simulink model "ASK_nc"  (R2020a)
settings: Solver=VariableStepDiscrete  StartTime=0.0  StopTime=tsim  RelTol=1e-3
values from neighbouring files (symbols this model uses):
  Ac = 1    [init_vars.m]
  B = rb    (= 1000)    [init_vars.m]
  fc = 10e3    (= 10000)    [init_vars.m]
  fs = spb * rb    (= 100000)    [init_vars.m]
  lim = 0.5/2    (= 0.25)    [parte3ASK.m]    (also in parte3BPSK.m = 0; parte4.m)
  rb = 1e3    (= 1000)    [init_vars.m]
  rng_seed = 5    [init_vars.m]
  spb = 100    [init_vars.m]
undefined symbols (not defined in the file or in its folder): fdesignblkfcn, gcbh
libraries: dspswit3 x2, commrandsrc3 x1, commchan3 x1, dspsigops x1, dspfdesign x1
settings Model: Creator=pedro  LastModifiedBy=pedro

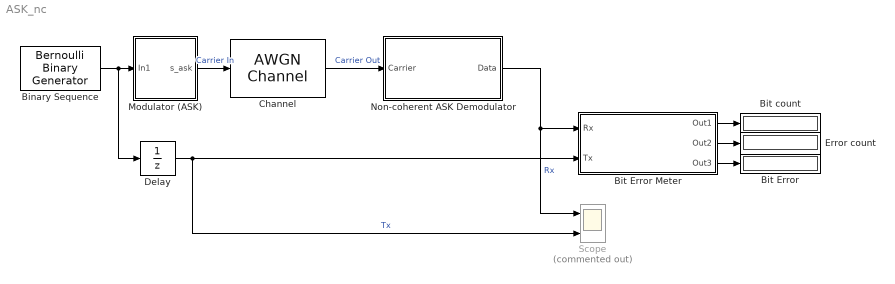
== system ASK_nc ==
  Binary Sequence : commrandsrc3/Bernoulli Binary Generator  ProbabilityOfZero=0.5  SeedSource=Parameter  Seed=rng_seed  SampleTime=1/rb  SamplesPerFrame=1  OutputDataType=double  SimulateUsing=Interpreted execution
  Bit Error : Display
  Bit Error Meter : Subsystem
  Bit count : Display
  Channel : commchan3/AWGN Channel  InputProcessing=Columns as channels (frame based)  seed=rng_seed  noiseMode=Variance from mask  EbNodB=10  EsNodB=10  SNRdB=10  bitsPerSym=1  Ps=1  Tsym=1  variance=sigmaquadrado
  Delay : UnitDelay  SampleTime=1/rb  HasFrameUpgradeWarning=on
  Error count : Display
  Modulator (ASK) : Subsystem
  Non-coherent ASK Demodulator : Subsystem
  Scope : Scope  Commented=on  NumInputPorts=2
  wires:
  Bit Error Meter/1(Out1) -> Bit count/1
  Bit Error Meter/2(Out2) -> Error count/1
  Delay/1 -> Scope/2, Bit Error Meter/2(Tx)  "Tx"
  Binary Sequence/1 -> Delay/1, Modulator (ASK)/1(In1)
  Bit Error Meter/3(Out3) -> Bit Error/1
  Modulator (ASK)/1(s_ask) -> Channel/1  "Carrier In"
  Channel/1 -> Non-coherent ASK Demodulator/1(Carrier)  "Carrier Out"
  Non-coherent ASK Demodulator/1(Data) -> Bit Error Meter/1(Rx), Scope/1  "Rx"

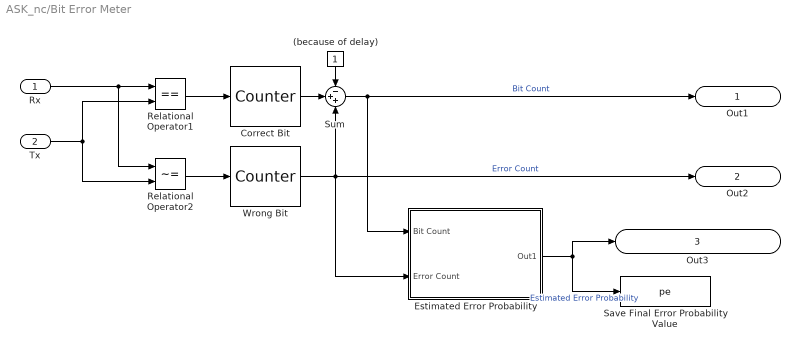
== system ASK_nc/Bit Error Meter ==
  Rx : Inport
  Tx : Inport  Port=2
  (because of delay) : Constant
  Correct Bit : dspswit3/Counter  Direction=Up  CountEvent=Non-zero sample  CounterSize=32 bits  MaxCount=255  InitialCount=0  Output=Count  HitValue=32  ResetInput=off  SamplesPerFrame=1  Ts=1  CntDtype=uint32  HitDtype=Logical
  Estimated Error Probability : Subsystem
  Relational Operator1 : RelationalOperator  Operator===  OutDataTypeStr=boolean  RndMeth=Simplest
  Relational Operator2 : RelationalOperator  Operator=~=  OutDataTypeStr=boolean  RndMeth=Simplest
  Save Final Error Probability Value : ToWorkspace  VariableName=pe  SampleTime=-1
      settings: MaxDataPoints=1
  Sum : Sum  Inputs=-++
  Wrong Bit : dspswit3/Counter  Direction=Up  CountEvent=Non-zero sample  CounterSize=32 bits  MaxCount=255  InitialCount=0  Output=Count  HitValue=32  ResetInput=off  SamplesPerFrame=1  Ts=1  CntDtype=uint32  HitDtype=Logical
  Out1 : Outport
  Out2 : Outport  Port=2
  Out3 : Outport  Port=3
  wires:
  Relational Operator1/1 -> Correct Bit/1
  Correct Bit/1 -> Sum/2
  Rx/1 -> Relational Operator2/1, Relational Operator1/1
  Relational Operator2/1 -> Wrong Bit/1
  Sum/1 -> Estimated Error Probability/1(Bit Count), Out1/1  "Bit Count"
  Tx/1 -> Relational Operator2/2, Relational Operator1/2
  Wrong Bit/1 -> Estimated Error Probability/2(Error Count), Sum/3, Out2/1  "Error Count"
  (because of delay)/1 -> Sum/1
  Estimated Error Probability/1(Out1) -> Save Final Error Probability Value/1, Out3/1  "Estimated Error Probability"

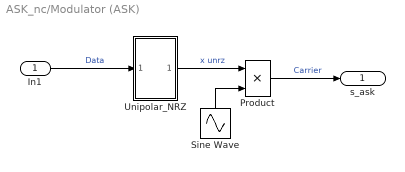
== system ASK_nc/Modulator (ASK) ==
  In1 : Inport
  Product : Product
  Sine Wave : Sin  Amplitude=Ac  Frequency=2*pi*fc  SampleTime=1/fs
  Unipolar_NRZ : Subsystem  mask(unipolar_nrz){Rb=rb, Spb=spb}
      mask prompts: Rb "Binary Data Rate"; Spb "Samples per bit"
  s_ask : Outport
  wires:
  Sine Wave/1 -> Product/2
  Product/1 -> s_ask/1  "Carrier"
  Unipolar_NRZ/1(Out1) -> Product/1  "x unrz"
  In1/1 -> Unipolar_NRZ/1(In1)  "Data"

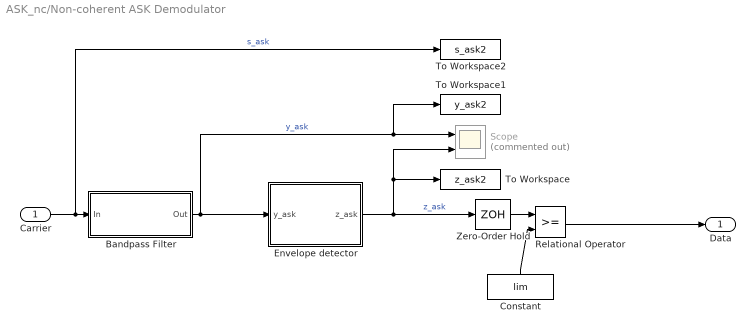
== system ASK_nc/Non-coherent ASK Demodulator ==
  Carrier : Inport
  Bandpass Filter : Subsystem  DialogController=fdesignblkfcn  InitFcn=fdesignblkfcn(gcbh, {'InitFcn'});  mask(Bandpass Filter){}
      mask help: Design a bandpass filter
      settings: CopyFcn=fdesignblkfcn(gcbh, {'CopyFcn'});
      mask Help: helpview(mapfilelocation('dsp'), 'dspbandpassfilter');
      mask Display: disp('Bandpass');
  Constant : Constant  Value=lim
  Envelope detector : Subsystem
  Relational Operator : RelationalOperator  OutDataTypeStr=boolean  RndMeth=Simplest
  Scope : Scope  Commented=on  NumInputPorts=2
  To Workspace : ToWorkspace  VariableName=z_ask2  SaveFormat=Timeseries  SampleTime=-1
  To Workspace1 : ToWorkspace  VariableName=y_ask2  SaveFormat=Timeseries  SampleTime=-1
  To Workspace2 : ToWorkspace  VariableName=s_ask2  SaveFormat=Timeseries  SampleTime=-1
  Zero-Order Hold : ZeroOrderHold  SampleTime=1/rb
  Data : Outport
  wires:
  Zero-Order Hold/1 -> Relational Operator/1
  Constant/1 -> Relational Operator/2
  Relational Operator/1 -> Data/1
  Envelope detector/1(z_ask) -> Scope/2, To Workspace/1, Zero-Order Hold/1  "z_ask"
  Bandpass Filter/1(Out) -> Envelope detector/1(y_ask), To Workspace1/1, Scope/1  "y_ask"
  Carrier/1 -> To Workspace2/1, Bandpass Filter/1(In)  "s_ask"

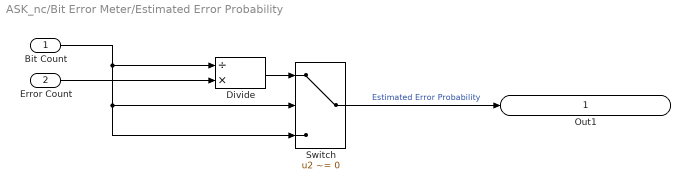
== system ASK_nc/Bit Error Meter/Estimated Error Probability ==
  Bit Count : Inport
  Error Count : Inport  Port=2
  Divide : Product  Inputs=/*  OutDataTypeStr=double
  Switch : Switch  Criteria=u2 ~= 0
  Out1 : Outport
  wires:
  Bit Count/1 -> Divide/1, Switch/3, Switch/2
  Switch/1 -> Out1/1  "Estimated Error Probability"
  Divide/1 -> Switch/1
  Error Count/1 -> Divide/2

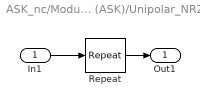
== system ASK_nc/Modulator (ASK)/Unipolar_NRZ ==
  In1 : Inport
  Repeat : dspsigops/Repeat  N=Spb  InputProcessing=Columns as channels (frame based)  RateOptions=Allow multirate processing  ic=0  mode=Unused parameter value
  Out1 : Outport
  wires:
  In1/1 -> Repeat/1
  Repeat/1 -> Out1/1

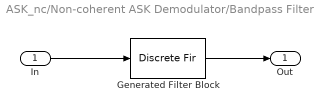
== system ASK_nc/Non-coherent ASK Demodulator/Bandpass Filter ==
  In : Inport
  Generated Filter Block : DiscreteFir  Tag=BlockMethodSubSystem  Coefficients=[0.0138126732487932231 0.0145041345154594357 0.00917515630259671186 -0.014886344687809314 -0.0580085472889965703 -0.0980336529237546134 -0.100786726198301022 -0.0459458005225757346 0.0518863238787333966 0.145858361924774721 0.184564824634511654 0.145858361924774721 0.0518863238787333966 -0.0459458005225757346 -0.100786726198301022 -0.0980336529237546134 -0.0580085472889965703 -0.014886344687809314 0.00917515630259671186 0.0145041345154594357 0.0138126732487932231]  InputProcessing=Columns as channels (frame based)
  Out : Outport  VectorParamsAs1DForOutWhenUnconnected=off
  wires:
  In/1 -> Generated Filter Block/1
  Generated Filter Block/1 -> Out/1

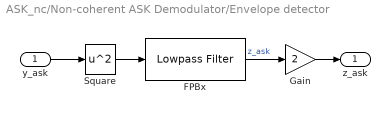
== system ASK_nc/Non-coherent ASK Demodulator/Envelope detector ==
  y_ask : Inport
  FPBx : dspfdesign/Lowpass Filter  FilterType=FIR  DesignForMinimumOrder=off  FilterOrder=20  PassbandFrequency=B  StopbandFrequency=B*(1+0.5)  PassbandRipple=0.1  StopbandAttenuation=80  InheritSampleRate=on  SampleRate=44100  SimulateUsing=Interpreted execution  roundingMode=Simplest  coeffsDataTypeStr=fixdt(1,16)
  Gain : Gain  Gain=2
  Square : Math  Operator=square  SaturateOnIntegerOverflow=on
  z_ask : Outport
  wires:
  y_ask/1 -> Square/1
  FPBx/1 -> Gain/1  "z_ask"
  Square/1 -> FPBx/1
  Gain/1 -> z_ask/1
